simulink model "WR_Control_LQR_Copy"  (R2019a)
settings: Solver=VariableStepAuto  StartTime=0.0  StopTime=5  RelTol=1e-6
undefined symbols (not defined in the file or in its folder): init
libraries: fuzblock x1
settings Model: Creator=phuon  LastModifiedBy=Duong
settings DataIOCC: ReturnWorkspaceOutputs=off
settings DebuggingCC: ArithmeticOperatorsInVariantConditions=warning
settings SFSimCC: SimUseLocalCustomCode=off
settings RTWCC: RTWUseLocalCustomCode=off

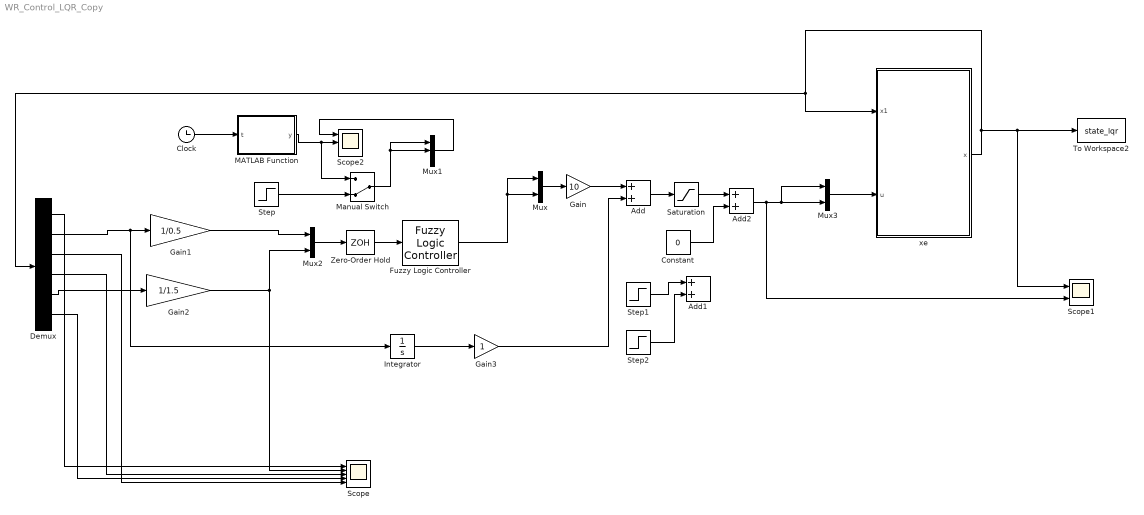
== system WR_Control_LQR_Copy ==
  Add : Sum
  Add1 : Sum
  Add2 : Sum
  Clock : Clock
  Constant : Constant  Value=0
  Demux : Demux  Outputs=6
  Fuzzy Logic Controller : fuzblock/Fuzzy Logic  Controller  FIS='1101ver5_sugeno.fis'  OutputSampleNumber=101  DataType=double  FuzzifiedInputs=off  RuleFiringStrengths=off  RuleOutputs=off  AggregatedOutputs=off  SimulateUsing=Interpreted execution  OutOfRangeInputValueMessage=warning  NoRuleFiredMessage=warning  EmptyOutputFuzzySetMessage=warning
  Gain : Gain  Gain=10
  Gain1 : Gain  Gain=1/0.5
  Gain2 : Gain  Gain=1/1.5
  Gain3 : Gain
  Integrator : Integrator
  MATLAB Function : MATLAB Function  TreatAsAtomicUnit=on
  Manual Switch : ManualSwitch  CurrentSetting=0
  Mux : Mux  Inputs=2
  Mux1 : Mux  Inputs=3
  Mux2 : Mux  Inputs=2
  Mux3 : Mux  Inputs=2
  Saturation : Saturate  UpperLimit=0.7  LowerLimit=-0.7
  Scope : Scope  NumInputPorts=5
  Scope1 : Scope  NumInputPorts=2
  Scope2 : Scope  NumInputPorts=3
  Step : Step  Time=0  After=0.01  SampleTime=0
  Step1 : Step  Time=2  After=0.7  SampleTime=0
  Step2 : Step  Time=2.5  After=-0.7  SampleTime=0
  To Workspace2 : ToWorkspace  VariableName=state_lqr  SaveFormat=Timeseries  SampleTime=-1
  Zero-Order Hold : ZeroOrderHold  SampleTime=1e-03
  "xe " : Subsystem
  wires:
  Demux/1 -> Scope/1
  Demux/3 -> Scope/5
  Demux/4 -> Scope/3
  Demux/5 -> Gain2/1
  Demux/6 -> Scope/4
  Fuzzy Logic Controller/1 -> Mux/2, Mux/1
  Mux/1 -> Gain/1
  MATLAB Function/1(y) -> Manual Switch/1, Scope2/2
  Clock/1 -> MATLAB Function/1(t)
  Manual Switch/1 -> Mux1/1, Mux1/2
  Step/1 -> Manual Switch/2
  Mux2/1 -> Zero-Order Hold/1
  Gain/1 -> Add/1
  Demux/2 -> Integrator/1, Gain1/1
  "xe "/1(x) -> Scope1/1, To Workspace2/1, Demux/1, "xe "/1(x1)
  Mux1/1 -> Scope2/1
  Gain1/1 -> Mux2/1
  Gain2/1 -> Scope/2, Mux2/2
  Mux3/1 -> "xe "/2(u)
  Add/1 -> Saturation/1
  Step1/1 -> Add1/1
  Step2/1 -> Add1/2
  Saturation/1 -> Add2/1
  Add2/1 -> Scope1/2, Mux3/1, Mux3/2
  Constant/1 -> Add2/2
  Integrator/1 -> Gain3/1
  Gain3/1 -> Add/2
  Zero-Order Hold/1 -> Fuzzy Logic Controller/1

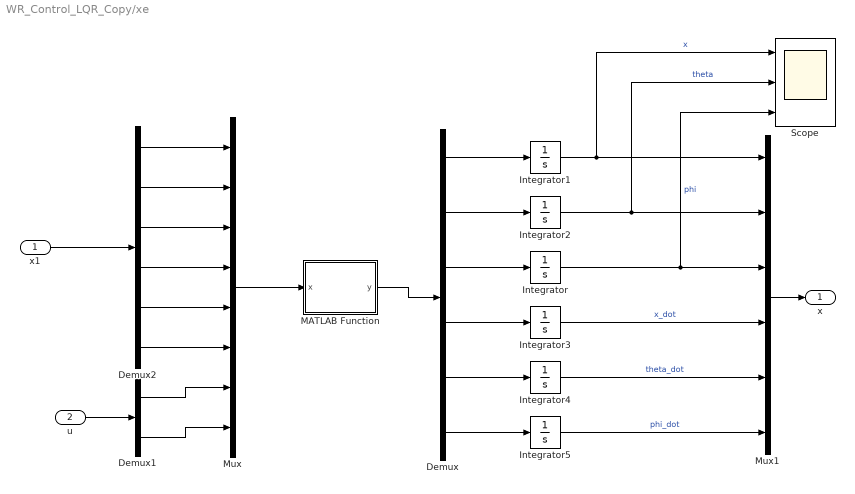
== system WR_Control_LQR_Copy/xe  ==
  x1 : Inport
  u : Inport  Port=2
  Demux : Demux  Outputs=6
  Demux1 : Demux  Outputs=2
  Demux2 : Demux  Outputs=6
  Integrator{,1,3..5} (5 alike) : Integrator
  Integrator2 : Integrator  InitialCondition=init
  MATLAB Function : MATLAB Function  TreatAsAtomicUnit=on
  Mux : Mux  Inputs=8
  Mux1 : Mux  Inputs=6
  Scope : Scope  NumInputPorts=3
  x : Outport
  wires:
  Demux/2 -> Integrator2/1
  Demux/3 -> Integrator/1
  Demux/6 -> Integrator5/1
  Demux/1 -> Integrator1/1
  Mux/1 -> MATLAB Function/1(x)
  MATLAB Function/1(y) -> Demux/1
  Demux/4 -> Integrator3/1
  Demux/5 -> Integrator4/1
  Demux1/1 -> Mux/7
  Demux1/2 -> Mux/8
  u/1 -> Demux1/1
  Integrator1/1 -> Scope/1, Mux1/1  "x"
  Integrator2/1 -> Scope/2, Mux1/2  "theta"
  Integrator/1 -> Mux1/3, Scope/3  "phi"
  Integrator3/1 -> Mux1/4  "x_dot"
  Integrator4/1 -> Mux1/5  "theta_dot"
  Integrator5/1 -> Mux1/6  "phi_dot"
  Mux1/1 -> x/1
  x1/1 -> Demux2/1
  Demux2/6 -> Mux/6
  Demux2/5 -> Mux/5
  Demux2/3 -> Mux/3
  Demux2/4 -> Mux/4
  Demux2/2 -> Mux/2
  Demux2/1 -> Mux/1

== matlab function WR_Control_LQR_Copy/xe /MATLAB Function ==
  data: x input; y output
function y = fcn(x)
y = zeros(6,1);
M = 0.765;
m = 0.03;
l = 0.10;
d =0.195;
r = 0.033;
%dong dien max: 
% Km=0.41202

I2 = M*l^2/2; %Momen quan tinh cua than xe doi voi goc theta
I3 = M*(d^2)/2; %Momen quan tinh cua than xe doi voi goc phi
I1 = I3;

J = m*r^2/2; %Momen quan tinh cua banh xe theo truc cua banh
K = m*r^2/4; %Momen quan tinh cua banh xe voi truc thang dung

g = 9.81;
C = 0.005;
x1 = x(1);
x2 = x(2);
x3 = x(3);
x4 = x(4); 
x5 = x(5);
x6 = x(6);
u1 = x(7);
u2 = x(8);
O1 = r^2*(M*l^2+I2)*((u1+u2)/r+2*C*(x5-x4/r)/r+M*l*sin(x2)*(x5^2+x6^2));
O2 = r^2*M*l*cos(x2)*(cos(x2)*sin(x2)*(I3-M*l^2-I1)*x6^2+(u1+u2)+2*C*(x5-x4/r)-M*l*g*sin(x2));
O3 = (2*J+(M+2*m)*r^2)*(cos(x2)*sin(x2)*(M*l^2+I1-I3)*x6^2-(u1+u2)-2*C*(x5-x4/r)+M*l*g*sin(x2));
O4 = -M*l*r^2*cos(x2)*((u1+u2)/r+2*C*(x5-x4/r)/r+M*l*sin(x2)*(x5^2+x6^2));
O5 = -2*r^2*(d*(u1-u2)/(2*r)+x6*sin(x2)*(M*l*x4+2*x5*cos(x2)*(M*l^2+I1-I3))+C*d^2*x6/(2*r^2));
O6 = r^2*(2*I3+4*K+m*d^2+2*(M*l^2+I1-I3)*(sin(x2))^2)+J*d^2;
O = (M*l*r)^2*(1-(cos(x2))^2)+2*I2*J+2*J*M*l^2+(I2*M+2*I2*m+2*M*m*l^2)*r^2;
y = [x4 x5 x6 (O1+O2)/O (O3+O4)/O O5/O6]';
end

== matlab function WR_Control_LQR_Copy/MATLAB Function ==
  data: t input; y output
function y = fcn(t)
% if t<0.07
%     y = 1;
% elseif (0.07<=t)&&(t<0.3)
%     y=-1;
% else
%     y=0;
y=-1;
end
